simulink subsystem "MAC"  (R2024a)
settings: Solver=VariableStepAuto  StartTime=0.0  StopTime=10.0  RelTol=1e-3
settings Model: Creator=versal  LastModifiedBy=versal

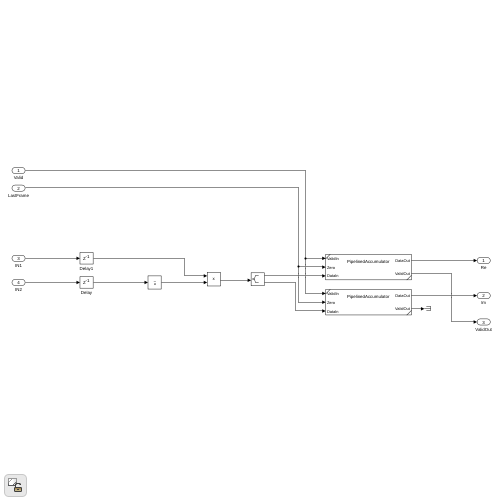
[thumbnail: Simulink's stored preview of the top-level diagram]
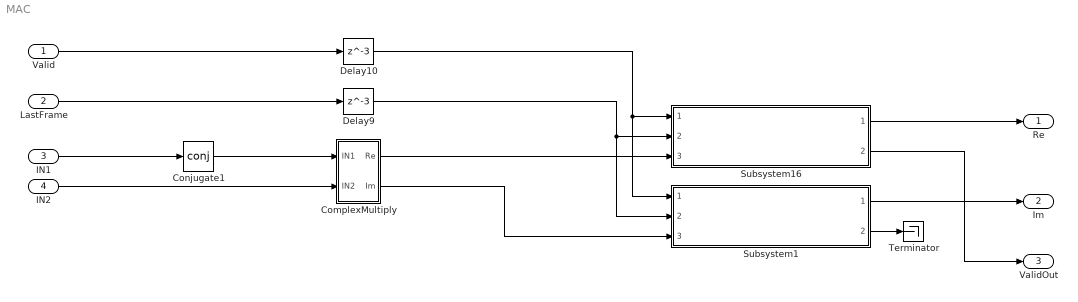
== system MAC ==
  Valid : Inport
  LastFrame : Inport  Port=2
  IN1 : Inport  Port=3
  IN2 : Inport  Port=4
  ComplexMultiply : Subsystem
  Conjugate1 : Math  Operator=conj  SignedPower=on  RndMeth=Zero
  Delay10 : Delay  DelayLength=3  InitialCondition=0  UseCircularBuffer=on
  Delay9 : Delay  DelayLength=3  InitialCondition=0  UseCircularBuffer=on
  Subsystem1 : Subsystem  ReferencedSubsystem=PipelinedAccumulator  PipelineLength=64
  Subsystem16 : Subsystem  ReferencedSubsystem=PipelinedAccumulator  PipelineLength=64
  Terminator : Terminator
  Re : Outport
  Im : Outport  Port=2
  ValidOut : Outport  Port=3
  wires:
  Subsystem16/1 -> Re/1
  Subsystem16/2 -> ValidOut/1
  Subsystem1/1 -> Im/1
  Subsystem1/2 -> Terminator/1
  Delay9/1 -> Subsystem16/2, Subsystem1/2
  LastFrame/1 -> Delay9/1
  Valid/1 -> Delay10/1
  IN1/1 -> Conjugate1/1
  IN2/1 -> ComplexMultiply/2(IN2)
  ComplexMultiply/2(Im) -> Subsystem1/3
  ComplexMultiply/1(Re) -> Subsystem16/3
  Delay10/1 -> Subsystem16/1, Subsystem1/1
  Conjugate1/1 -> ComplexMultiply/1(IN1)

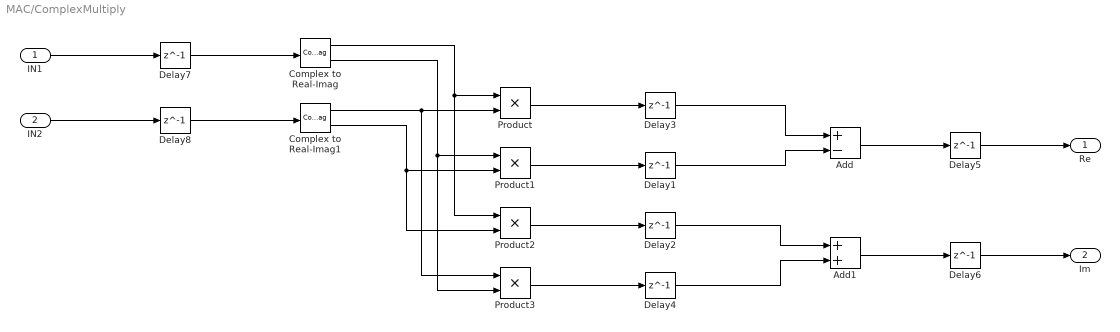
== system MAC/ComplexMultiply ==
  IN1 : Inport
  IN2 : Inport  Port=2
  Add : Sum  Inputs=+-
  Add1 : Sum
  Complex to Real-Imag : ComplexToRealImag
  Complex to Real-Imag1 : ComplexToRealImag
  Delay{1..8} (8 alike) : Delay  DelayLength=1  InitialCondition=0  UseCircularBuffer=on
  Product{,1..3} (4 alike) : Product
  Re : Outport
  Im : Outport  Port=2
  wires:
  Delay8/1 -> Complex to Real-Imag1/1
  Delay7/1 -> Complex to Real-Imag/1
  Delay6/1 -> Im/1
  Delay5/1 -> Re/1
  Add/1 -> Delay5/1
  Add1/1 -> Delay6/1
  Delay4/1 -> Add1/2
  Delay2/1 -> Add1/1
  Delay1/1 -> Add/2
  Delay3/1 -> Add/1
  Product1/1 -> Delay1/1
  Product2/1 -> Delay2/1
  Product3/1 -> Delay4/1
  Complex to Real-Imag1/2 -> Product2/2, Product1/2
  Complex to Real-Imag1/1 -> Product/2, Product3/1
  Complex to Real-Imag/2 -> Product3/2, Product1/1
  Complex to Real-Imag/1 -> Product/1, Product2/1
  IN2/1 -> Delay8/1
  IN1/1 -> Delay7/1
  Product/1 -> Delay3/1
